simulink model "PV-battery(2)"  (R2018a)
settings: Solver=ode15s  StartTime=0.0  StopTime=0.8  MaxStep=1e-4  RelTol=1e-2
undefined symbols (not defined in the file): BMSS, Ion, Lithium
libraries: powerlib x19, powerlib_extras x2, electricdrivelib x1, fuzblock x1, re_lib x1, powerlib_meascontrol x1
settings Model: Creator=venka  LastModifiedBy=Yasser-PC
settings SolverCC: ZeroCrossControl=DisableAll  InsertRTBMode=Always
settings CodeAppCC: StateflowObjectComments=on
settings SimscapeCC: SimscapeNormalizeSystem=off

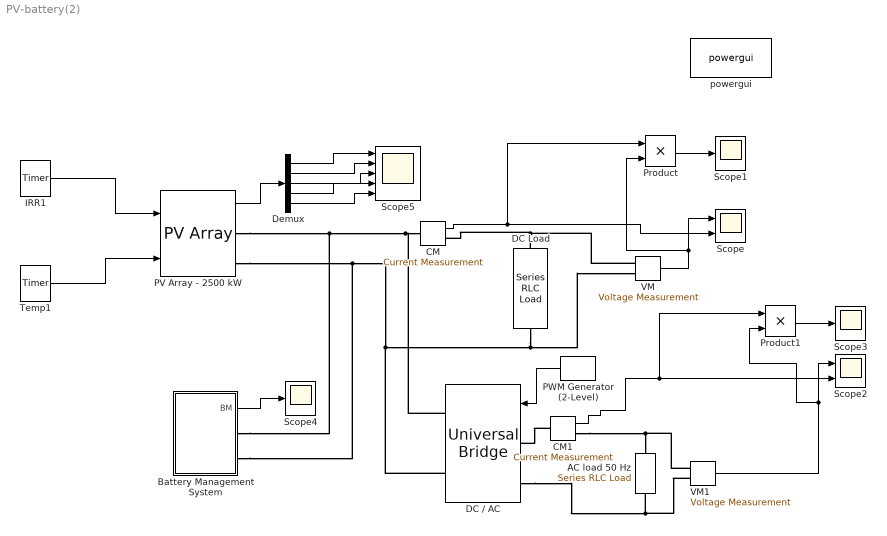
== system PV-battery(2) ==
  AC load 50 Hz : powerlib/Elements/Series RLC Load  LConnTagsString=a  RConnTagsString=__new0  NominalVoltage=220  NominalFrequency=50  ActivePower=10e3  InductivePower=0  CapacitivePower=0  Setx0=off  InitialVoltage=0  SetiL0=off  InitialCurrent=0  Measurements=None  LoadType=constant Z
  Battery Management System : Subsystem
  CM : powerlib/Measurements/Current Measurement  PhasorSimulation=off  OutputType=Complex  PSBequivalent=0
  CM1 : powerlib/Measurements/Current Measurement  PhasorSimulation=off  OutputType=Complex  PSBequivalent=0
  DC / AC : powerlib/Power Electronics/Universal Bridge  Arms=2  SnubberResistance=1e5  SnubberCapacitance=inf  Device=MOSFET / Diodes  Ron=1e-3  Lon=0  ForwardVoltages="[  0  0  ]"  ForwardVoltage=0  GTOparameters=[ 10e-6 , 20e-6 ]  IGBTparameters=[ 1e-6 , 2e-6 ]  Measurements=None  Measurements_2=None  converterType=Rectifier
  "DC Load " : powerlib/Elements/Series RLC Load  LConnTagsString=a  RConnTagsString=__new0  NominalVoltage=220  NominalFrequency=0.0001  ActivePower=5e3  InductivePower=0  CapacitivePower=0  Setx0=off  InitialVoltage=0  SetiL0=off  InitialCurrent=0  Measurements=None  LoadType=constant Z
  Demux : Demux  Outputs=5
  IRR1 : powerlib_extras/Control  Blocks/Timer  t=[0 0.2 0.4 0.5 0.6]  e=[500 700 900 1000 100]
  PV Array - 2500 kW : re_lib/Solar/PV Array  Npar=10  Nser=1  PlotType=array @ 25 deg.C & specified irradiances  S_vec="[ 1000  500  250 ]"  Temp_C_vec="[ 45 25  ]"  ModuleName=American Solar Wholesale ASW-250P  PlotWhenSelected=off  Pm=249.92  Ncell=72  Voc=43.22  Isc=7.76  Vm=35.2  Im=7.1  beta_Voc_pc=-0.3028  alpha_Isc_pc=0.035271  beta_Voc=-0.13087  alpha_Isc=0.002737  IL=7.7892  I0=2.8649e-11  nI=0.88912  Rsh=111.8766  Rs=0.42122  BAL=off  Tc=1e-6  Tfilter=5e-6
  PWM Generator (2-Level) : powerlib_meascontrol/Pulse & Signal Generators/PWM Generator (2-Level)  ModulatorType=Single-phase full-bridge (4 pulses)  ModulatorMode=Unsynchronized  Fc=27*60  Pc=90  nF=27  MinMax="[ -1  1 ]"  SamplingTechnique=Natural  ModulatingSignals=on  m=0.8  Freq=50  Phase=0  Ts=0  ShowCarrierOutport=off
      settings: SourceProductName=Simscape Power Systems
  Product : Product
  Product1 : Product
  Scope : Scope  NumInputPorts=2
  Scope1 : Scope
  Scope2 : Scope  NumInputPorts=2
  Scope3 : Scope
  Scope4 : Scope
  Scope5 : Scope  NumInputPorts=5
  Temp1 : powerlib_extras/Control  Blocks/Timer  t=[0 0.2 0.4 0.5 0.6]  e=[20 23 25 28 25]
  VM : powerlib/Measurements/Voltage Measurement  PhasorSimulation=off  OutputType=Complex  PSBequivalent=0
  VM1 : powerlib/Measurements/Voltage Measurement  PhasorSimulation=off  OutputType=Complex  PSBequivalent=0
  powergui : powerlib/powergui  Priority=1  SimulationMode=Discrete  SampleTime=1e-8  frequency=60  Iterations=50  frequencyindice=0  Pbase=100e6  ErrMax=1e-4  UnitsV=kV  UnitsW=MW  buscounter=0  FunctionMessages=on  echomessages=on  EnableUseOfTLC=on  CurrentSourceSwitches=off  DisableSnubberDevices=off  DisableRonSwitches=off  DisableVfSwitches=off  DisplayEquations=off  SolverType=Backward Euler  Interpol=off  ExternalGateDelay=off  methode=off  Ts=100  x0status=steady  SPID=on  SwTol=0  HookPort=off  RestoreLinks=warning  ResistiveCurrentMeasurement=off  Frange=[0:2:500]  Ylog=off  Xlog=on  ShowGrid=off  save=off  variable=ZData  structure=0  ZoomFFT=off  StartTime=0.0  cycles=1  DisplayStyle=1  fundamental=60  FreqAxis=off  MaxFrequency=1000  frequencyindicesteady=1  RmsSteady=1  display=off
  wires:
  VM/1 -> Product/2, Scope/1
  CM/1 -> Product/1, Scope/2
  Product/1 -> Scope1/1
  VM1/1 -> Product1/2, Scope2/1
  CM1/1 -> Product1/1, Scope2/2
  Product1/1 -> Scope3/1
  PWM Generator (2-Level)/1 -> DC / AC/1
  Battery Management System/1("BM ") -> Scope4/1
  Temp1/1 -> PV Array - 2500 kW/2
  IRR1/1 -> PV Array - 2500 kW/1
  PV Array - 2500 kW/1 -> Demux/1
  Demux/1 -> Scope5/1
  Demux/2 -> Scope5/2
  Demux/3 -> Scope5/3
  Demux/4 -> Scope5/4
  Demux/5 -> Scope5/5
  connections:
  PV Array - 2500 kW/RConn2 -- Battery Management System/RConn2 -- DC / AC/RConn2 -- "DC Load "/RConn1 -- VM/LConn2
  PV Array - 2500 kW/RConn1 -- Battery Management System/RConn1 -- DC / AC/RConn1 -- CM/LConn1
  "DC Load "/LConn1 -- VM/LConn1 -- CM/RConn1
  CM1/LConn1 -- DC / AC/LConn1
  DC / AC/LConn2 -- AC load 50 Hz/RConn1 -- VM1/LConn2
  CM1/RConn1 -- VM1/LConn1 -- AC load 50 Hz/LConn1

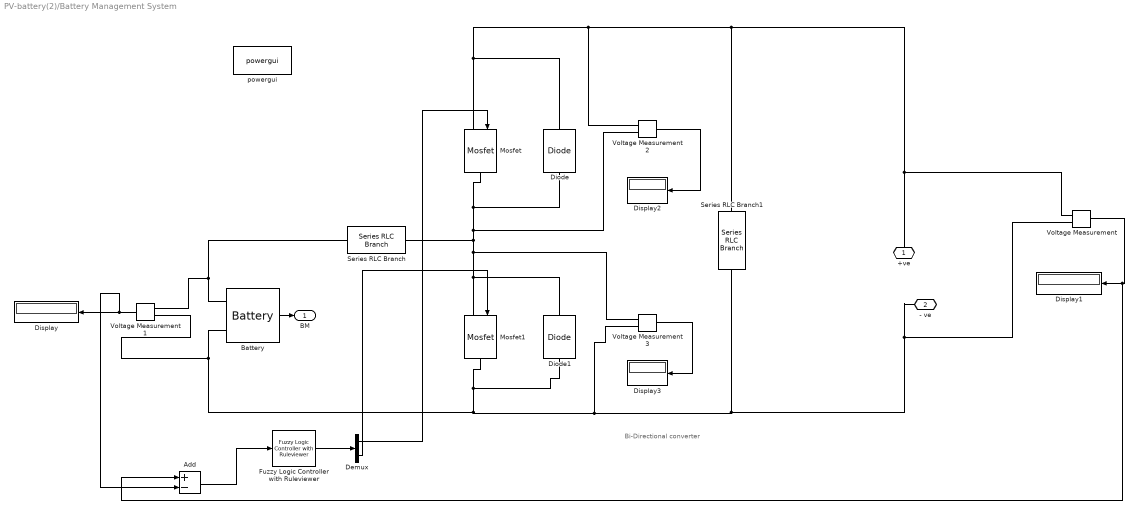
== system PV-battery(2)/Battery Management System ==
  note: Bi-Directional converter
  Add : Sum  Inputs=+-
  Battery : electricdrivelib/Extra Sources/Battery  BatType=Lithium-Ion  ShowTempParam=off  ThermalPreset=no  ShowAgeParam=off  NomV=12  NomQ=100  SOC=100  Batt_Tr=0.1  PresetModel=off  MaxQ=50  MinV=180  FullV=220  Dis_rate=45  R=0.013333  Normal_OP=220  expZone="[220      40]"  current=[40 45 50]  Units=Time  Tci=20  NomT=20  T2=-30  MaxQ2=4.8  FullV2=7.1  Normal_OP2=5.655  expZone2="[6.58           1]"  Rca=0.6  ti=2000  Dp=0  Neq0=0  Tsim=1e6  Ta1=25  Qeol=5.4*0.9  Reol=0.013333*1.2  Char_age=[2.3478, 3]  Dis_age=[2.3478, 10]  N1=1500  N2=10500  N3=1000  N4=1400  Ta2=45  N5=950
  Demux : Demux  Outputs=2
  Diode : powerlib/Power Electronics/Diode  Ron=0.001  Lon=0  Vf=0.8  IC=0  UseSnubber=0  Rs=500  Cs=250e-9  Measurements=off
  Diode1 : powerlib/Power Electronics/Diode  Ron=0.001  Lon=0  Vf=0.8  IC=0  UseSnubber=0  Rs=500  Cs=250e-9  Measurements=off
  Display{,1..3} (4 alike) : Display
  Fuzzy Logic Controller with Ruleviewer : fuzblock/Fuzzy Logic  Controller  with Ruleviewer  fismatrix=[BMSS]  Ts=0.1
  Mosfet : powerlib/Power Electronics/Mosfet  Ron=0.1  Lon=0  Rd=0.01  Vfd=0  IC=0  Rs=1e5  Cs=inf  Measurements=off
  Mosfet1 : powerlib/Power Electronics/Mosfet  Ron=0.1  Lon=0  Rd=0.01  Vfd=0  IC=0  Rs=1e5  Cs=inf  Measurements=off
  Series RLC Branch : powerlib/Elements/Series RLC Branch  LConnTagsString=__new0  RConnTagsString=__new0  BranchType=L  Resistance=1  Inductance=1e-3  SetiL0=off  InitialCurrent=0  Capacitance=1e-6  Setx0=off  InitialVoltage=0  Measurements=None
  Series RLC Branch1 : powerlib/Elements/Series RLC Branch  LConnTagsString=__new0  RConnTagsString=__new0  BranchType=RC  Resistance=1  Inductance=1e-3  SetiL0=off  InitialCurrent=0  Capacitance=1e-6  Setx0=off  InitialVoltage=0  Measurements=None
  Voltage Measurement{,1..3} (4 alike) : powerlib/Measurements/Voltage Measurement  PhasorSimulation=off  OutputType=Complex  PSBequivalent=0
  powergui : powerlib/powergui  Priority=1  SimulationMode=Continuous  SampleTime=50e-6  frequency=60  Iterations=50  frequencyindice=0  Pbase=100e6  ErrMax=1e-4  UnitsV=kV  UnitsW=MW  buscounter=0  FunctionMessages=off  echomessages=off  EnableUseOfTLC=off  CurrentSourceSwitches=off  DisableSnubberDevices=off  DisableRonSwitches=off  DisableVfSwitches=off  DisplayEquations=off  SolverType=Tustin/Backward Euler (TBE)  Interpol=off  ExternalGateDelay=off  methode=off  Ts=100  x0status=blocks  SPID=on  SwTol=0  HookPort=off  RestoreLinks=warning  ResistiveCurrentMeasurement=off  Frange=[0:2:500]  Ylog=off  Xlog=on  ShowGrid=off  save=off  variable=ZData  structure=0  ZoomFFT=off  StartTime=0.0  cycles=1  DisplayStyle=1  fundamental=60  FreqAxis=off  MaxFrequency=1000  frequencyindicesteady=1  RmsSteady=1  display=off
  +ve : PMIOPort  Side=Right
  - ve : PMIOPort  Port=2  Side=Right
  "BM " : Outport
  wires:
  Voltage Measurement3/1 -> Display3/1
  Voltage Measurement2/1 -> Display2/1
  Voltage Measurement1/1 -> Add/2, Display/1
  Voltage Measurement/1 -> Add/1, Display1/1
  Battery/1 -> "BM "/1
  Fuzzy Logic Controller with Ruleviewer/1 -> Demux/1
  Demux/1 -> Mosfet/1
  Add/1 -> Fuzzy Logic Controller with Ruleviewer/1
  Demux/2 -> Mosfet1/1
  connections:
  Mosfet/RConn1 -- Diode/LConn1 -- Voltage Measurement2/LConn2 -- Series RLC Branch/RConn1 -- Voltage Measurement3/LConn1 -- Diode1/RConn1 -- Mosfet1/LConn1
  Voltage Measurement1/LConn1 -- Series RLC Branch/LConn1 -- Battery/LConn1
  Mosfet/LConn1 -- Diode/RConn1 -- Voltage Measurement2/LConn1 -- Series RLC Branch1/LConn1 -- Voltage Measurement/LConn1 -- +ve/RConn1
  Mosfet1/RConn1 -- Diode1/LConn1 -- Battery/LConn2 -- Voltage Measurement1/LConn2 -- Voltage Measurement3/LConn2 -- Series RLC Branch1/RConn1 -- Voltage Measurement/LConn2 -- - ve/RConn1
